simulink model "FLC"  (R2022b)
settings: Solver=VariableStepAuto  StartTime=0.0  StopTime=180  RelTol=1e-3
undefined symbols (not defined in the file or in its folder): sigbuilder_block
settings Model: Creator=ztall  LastModifiedBy=ztall

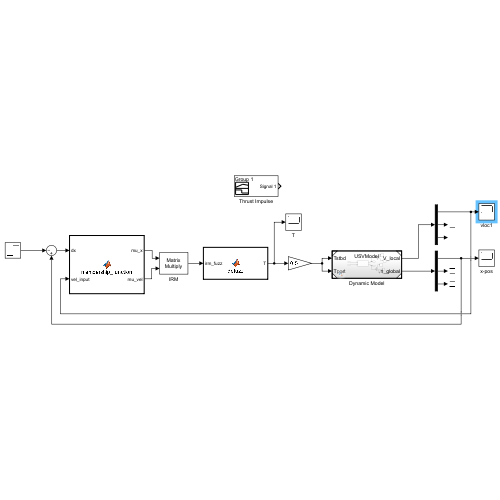
[thumbnail: Simulink's stored preview of the top-level diagram]
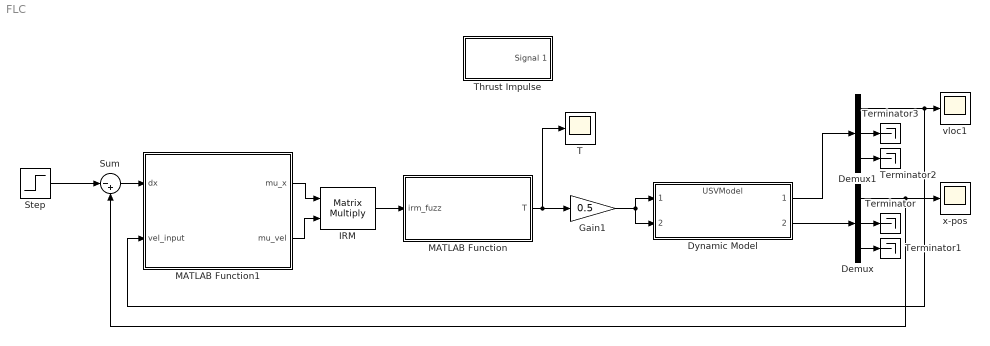
== system FLC ==
  Demux : Demux  Outputs=3
  Demux1 : Demux  Outputs=3
  Dynamic Model : ModelReference  ModelNameDialog=USVModel.slx  SimulationMode=Normal  ModelReferenceVersion=7.1
  Gain1 : Gain  Gain=0.5
  IRM : Product  Multiplication=Matrix(*)
  MATLAB Function : MATLAB Function  TreatAsAtomicUnit=on
  MATLAB Function1 : MATLAB Function  TreatAsAtomicUnit=on
  Step : Step  Time=5  After=15  SampleTime=0
  Sum : Sum  Inputs=|-+
  T : Scope
  Terminator{,1..3} (4 alike) : Terminator
  Thrust Impulse : Subsystem  Tag=STV Subsys  LoadFcn=sigbuilder_block('load');  StartFcn=sigbuilder_block('start');  StopFcn=sigbuilder_block('stop');  ClipboardFcn=sigbuilder_block('clipboard');  mask(Sigbuilder block){tuvar=[0:10]}
      mask help: Simulink:masks:SigbuilderBlock_MD
      mask init:
      | if ~strcmp(get_param(bdroot(gcbh),'SimulationStatus'),'stopped') tuvar = sigbuilder_block('maskInit'); end
      settings: CopyFcn=sigbuilder_block('copy');  DeleteFcn=sigbuilder_block('delete');  ModelCloseFcn=sigbuilder_block('modelClose');  PreSaveFcn=sigbuilder_block('preSave');  PauseFcn=sigbuilder_block('pause');  ContinueFcn=sigbuilder_block('continue');  NameChangeFcn=sigbuilder_block('namechange');  OpenFcn=sigbuilder_block('open',[437.6 199.2 550.4 400 ]);  CloseFcn=sigbuilder_block('close');
      mask Display: plot(0, 0, 100, 100,[2, 2, 32, 32, 2], [68, 8, 8, 68, 68],[32, 2], [38, 38], [32, 19, 2],[53, 60, 44], [32, 17, 17, 2],[16, 16, 31, 31]);txt = getActiveGroup(gcbh);text(2, 100, txt,'verticalAlignment', 'top');
  vloc1 : Scope
  x-pos : Scope
  wires:
  Sum/1 -> MATLAB Function1/1(dx)
  MATLAB Function1/1(mu_x) -> IRM/1
  MATLAB Function1/2(mu_vel) -> IRM/2
  IRM/1 -> MATLAB Function/1(irm_fuzz)
  MATLAB Function/1(T) -> Gain1/1, T/1
  Dynamic Model/2 -> Demux/1
  Demux/3 -> Terminator1/1
  Dynamic Model/1 -> Demux1/1
  Demux1/1 -> MATLAB Function1/2(vel_input), vloc1/1
  Demux/2 -> Terminator/1
  Demux/1 -> x-pos/1, Sum/2
  Step/1 -> Sum/1
  Demux1/2 -> Terminator3/1
  Demux1/3 -> Terminator2/1
  Gain1/1 -> Dynamic Model/1, Dynamic Model/2

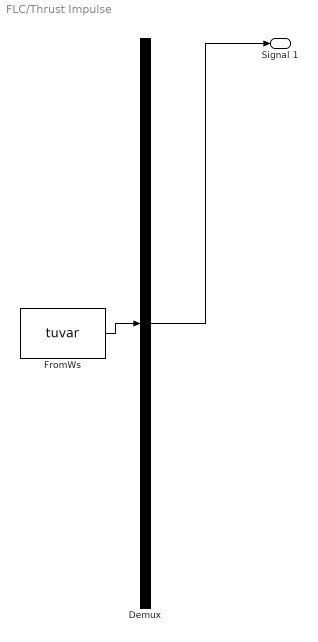
== system FLC/Thrust Impulse ==
  Demux : Demux  Tag=STV Demux  Outputs=1
      settings: DisplayOption=none
  FromWs : FromWorkspace  Tag=STV FromWs  VariableName=tuvar
      SigBuilderData=|
      | common.afterFinalStr = 'Extrapolate'
      | common.sampleTime = 0
      | dataSet.timeRange = [0 10]
      | dataSet.name = 'Group 1'
      | sbobj.Groups.Name = 'Group 1'
      | sbobj.Groups.Signals.Name = 'Signal 1'
      | sbobj.Groups.Signals.XData = [0 2 2 3.04 3.04 10]
      | sbobj.Groups.Signals.YData = [-0.005 0 20 20 0 0]
  Signal 1 : Outport  Tag=STV Outport
  wires:
  Demux/1 -> Signal 1/1
  FromWs/1 -> Demux/1

== matlab function FLC/MATLAB Function ==
  data: irm_fuzz input; T output
function T = defuzz(irm_fuzz)

%trapezoid base sizes
LB = 300;
SB = 100;

%area calulcations
area_mat = zeros(5,5);

a = 1;
b = 1;

while a < 6
    while b < 6
        area_mat(a,b) = LB*irm_fuzz(a,b) - (((irm_fuzz(a,b))^2)/2)*(LB - SB);
        b = b + 1;
        
    end
    b = 1;
    a = a + 1;
end

%centroids
CLN = -300;
CN = -150;
CZ = 0;
CP = 150;
CLP = 300;

cent_mat = [CLP,CLP,CP,CP, CZ;...
            CLP,CP, CP,CZ, CN;...
            CP, CP, CZ,CN, CN;...
            CP, CZ, CN,CN, CLN;...
            CZ, CN, CN,CLN,CLN];

%summation
%centroid*area
numerator = 0;
a = 1;
b = 1;
while a < 6
    while b < 6
        numerator = numerator + area_mat(a,b)*cent_mat(a,b);
        b = b + 1;
        
    end
    b = 1;
    a = a + 1;
end

%denominator
a = 1;
b = 1;
denom = 0;
while a < 6
    while b < 6
        denom = denom + area_mat(a,b);
        
        b = b + 1;
        
    end
    b = 1;
    a = a + 1;
end

T = numerator/denom;

end

== matlab function FLC/MATLAB Function1 ==
  data: dx input; mu_x output; vel_input input; mu_vel output
function [mu_x,mu_vel] = membership_function(dx,vel_input)
%Membership functions for the linguistic values of position error and
%velocity
%mu_x and mu_vel contains the following values (in order):
%  mu_* = [LN,N,Z,P,LP]
mu_x = zeros(5,1);
%% Position Error

% large negative (LN)
if dx <= -15
    mu_x(1) = 1;
elseif dx > -15 && dx <= -9
    mu_x(1) = -1/6*dx-3/2;
else
    mu_x(1) = 0;
end

% negative (N)
if dx >= -12 && dx <= -6
    mu_x(2) = 1;
elseif dx >= -18 && dx < -12
    mu_x(2) = 1/6*dx+3;
elseif dx > -6 && dx <= 0
    mu_x(2) = -1/6*dx;
else
    mu_x(2) = 0;
end

% zero
if dx >= -3 && dx <= 3
    mu_x(3) = 1;
elseif dx >= -9 && dx < -3
    mu_x(3) = 1/6*dx+3/2;
elseif dx > 3 && dx <= 9
    mu_x(3) = -1/6*dx+3/2;
else
    mu_x(3) = 0;
end

% positive
if dx >= 6 && dx <= 12
    mu_x(4) = 1;
elseif dx >= 0 && dx < 6
    mu_x(4) = 1/6*dx;
elseif dx > 12 && dx <= 18
    mu_x(4) = -1/6*dx+3;
else
    mu_x(4) = 0;
end

% large positive
if dx >= 15
    mu_x(5) = 1;
elseif dx > 9 && dx <= 15
    mu_x(5) = 1/6*dx-3/2;
else
    mu_x(5) = 0;
end

%% Velocity

% large negative (LN)
if vel_input < -7
    mu_vel = [1,0,0,0,0];

elseif vel_input < -5
    LN = (-1/2*vel_input)-5/2;
    N = (1/2*vel_input)+7/2;
    mu_vel = [LN,N,0,0,0];
    
% negative (N)
elseif vel_input < -3
    mu_vel = [0,1,0,0,0];
    
elseif vel_input < -1
    N = (-1/2*vel_input)-1/2;
    Z = (1/2*vel_input)+3/2;
    mu_vel = [0,N,Z,0,0];

% zero (Z)
elseif vel_input < 1
    mu_vel = [0,0,1,0,0];
    
elseif vel_input < 3
    Z = (-1/2*vel_input)+3/2;
    P = (1/2*vel_input)-1/2;
    mu_vel = [0,0,Z,P,0];
    
%positive (P)   
elseif vel_input < 5
    mu_vel = [0,0,0,1,0];
    
elseif vel_input < 7
    P = (-1/2*vel_input)+7/2;
    L = (1/2*vel_input)-5/2;
    mu_vel = [0,0,0,P,L];
    
%large positive (LP)
else
    mu_vel = [0,0,0,0,1];
    
end

end
